simulink library "LumArduinoMAX31856"  (R2024a)
settings: Solver=VariableStepAuto  StartTime=0.0  StopTime=10.0  RelTol=1e-3
undefined symbols (not defined in the file or in its folder): deltaT_s, MAX31856_CJTH_REG_READ, MAX31856_CJTL_REG_READ, MAX31856_CJTO_REG_READ, MAX31856_CJTO_REG_WRITE, MAX31856_CR0_REG_READ, MAX31856_CR0_REG_WRITE, MAX31856_CR1_REG_READ, MAX31856_CR1_REG_WRITE, MAX31856_LTCBH_REG_READ, MAX31856_LTCBL_REG_READ, MAX31856_LTCBM_REG_READ, MAX31856_MASK_REG_WRITE, pin_CS
libraries: arduinolib x12, LumArduino x8
settings Model: Creator=chris  LastModifiedBy=chris

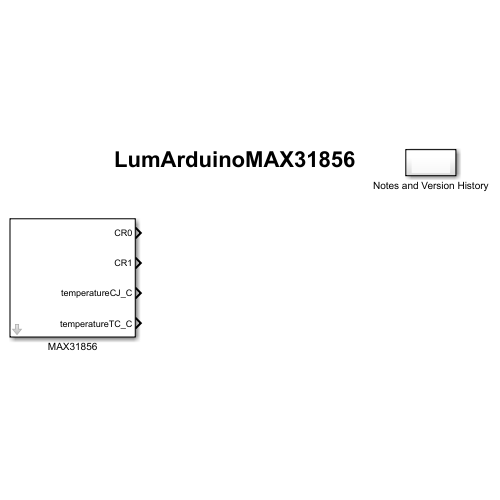
[thumbnail: Simulink's stored preview of the top-level diagram]
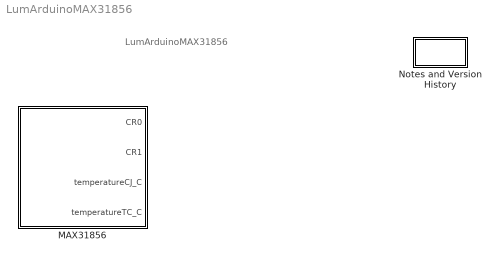
== system LumArduinoMAX31856 ==
  note: LumArduinoMAX31856
  MAX31856 : Subsystem  mask{MAX31856_CR0_REG_READ=MAX31856_CR0_REG_READ, MAX31856_CR0_REG_WRITE=MAX31856_CR0_REG_WRITE, MAX31856_CR1_REG_READ=MAX31856_CR1_REG_READ, MAX31856_CR1_REG_WRITE=MAX31856_CR1_REG_WRITE, MAX31856_MASK_REG_WRITE=MAX31856_MASK_REG_WRITE, MAX31856_CJTO_REG_READ=MAX31856_CJTO_REG_READ, MAX31856_CJTO_REG_WRITE=MAX31856_CJTO_REG_WRITE, MAX31856_CJTH_REG_READ=MAX31856_CJTH_REG_READ, MAX31856_CJTL_REG_READ=MAX31856_CJTL_REG_READ, MAX31856_LTCBH_REG_READ=MAX31856_LTCBH_REG_READ, MAX31856_LTCBM_REG_READ=MAX31856_LTCBM_REG_READ, MAX31856_LTCBL_REG_READ=MAX31856_LTCBL_REG_READ, deltaT_s=deltaT_s, pin_CS=pin_CS}
      mask prompts: MAX31856_CR0_REG_READ "CR0 Read Register Address"; MAX31856_CR0_REG_WRITE "CR0 Write Register Address"; MAX31856_CR1_REG_READ "CR1 Read Register Address"; MAX31856_CR1_REG_WRITE "CR1 Write Register Address"; MAX31856_MASK_REG_WRITE "MASK Write Register Address"; MAX31856_CJTO_REG_READ "CJTO Read Register Address"; MAX31856_CJTO_REG_WRITE "CJTO Write Register Address"; MAX31856_CJTH_REG_READ "CJTH Read Register Address"; MAX31856_CJTL_REG_READ "CJTL Read Register Address"; MAX31856_LTCBH_REG_READ "LTCBH Read Register Address"; MAX31856_LTCBM_REG_READ "LTCBM Read Register Address"; MAX31856_LTCBL_REG_READ "LTCBL Read Register Address"; deltaT_s "Sample Time (sec)"; pin_CS "Chip Select Pin"
      mask help:
      | Interface with a MAX31856 breakout board.
      |
      | Currently this only supports K-type thermocouples.
      |
      | Christopher Lum
      | lum@uw.edu
      mask DialogControl ParameterGroupVar Prompt: CR0
      mask DialogControl Container3 Prompt: CR1
      mask DialogControl Container5 Prompt: MASK
      mask DialogControl Container4 Prompt: CJTO
      mask DialogControl Container6 Prompt: CJTL/CJTH
      mask DialogControl Container7 Prompt: LTCBH/LTCBM/LTCBL
      mask DialogControl Container8 Prompt: Misc.
  Notes and Version History : Subsystem

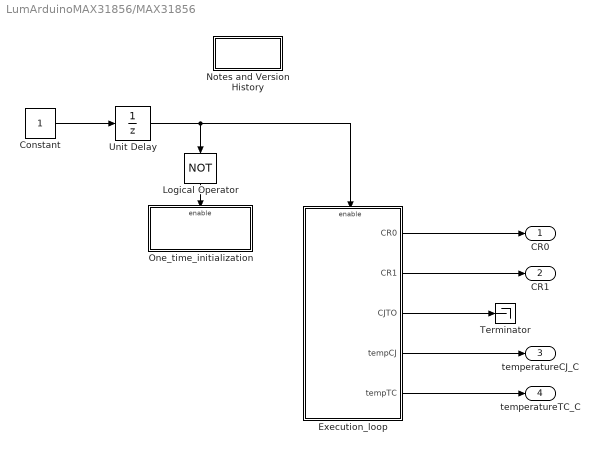
== system LumArduinoMAX31856/MAX31856 ==
  Constant : Constant  OutDataTypeStr=boolean  SampleTime=deltaT_s
  Execution_loop : Subsystem  TreatAsAtomicUnit=on
  Logical Operator : Logic  Operator=NOT  AllPortsSameDT=off  OutDataTypeStr=boolean
  Notes and Version History : Subsystem
  One_time_initialization : Subsystem  TreatAsAtomicUnit=on
  Terminator : Terminator
  Unit Delay : UnitDelay  SampleTime=-1  HasFrameUpgradeWarning=on
  CR0 : Outport
  CR1 : Outport  Port=2
  temperatureCJ_C : Outport  Port=3
  temperatureTC_C : Outport  Port=4
  wires:
  Execution_loop/4(tempCJ) -> temperatureCJ_C/1
  Execution_loop/5(tempTC) -> temperatureTC_C/1
  Execution_loop/3(CJTO) -> Terminator/1
  Execution_loop/2(CR1) -> CR1/1
  Logical Operator/1 -> One_time_initialization/Enable
  Execution_loop/1(CR0) -> CR0/1
  Unit Delay/1 -> Logical Operator/1, Execution_loop/Enable
  Constant/1 -> Unit Delay/1

== system LumArduinoMAX31856/Notes and Version History ==
  note: Interfacing with the MAX31856 sensor
      |
      | Christopher Lum
      | lum@uw.edu
      |
      | Version History
      | 01/04/25: Created

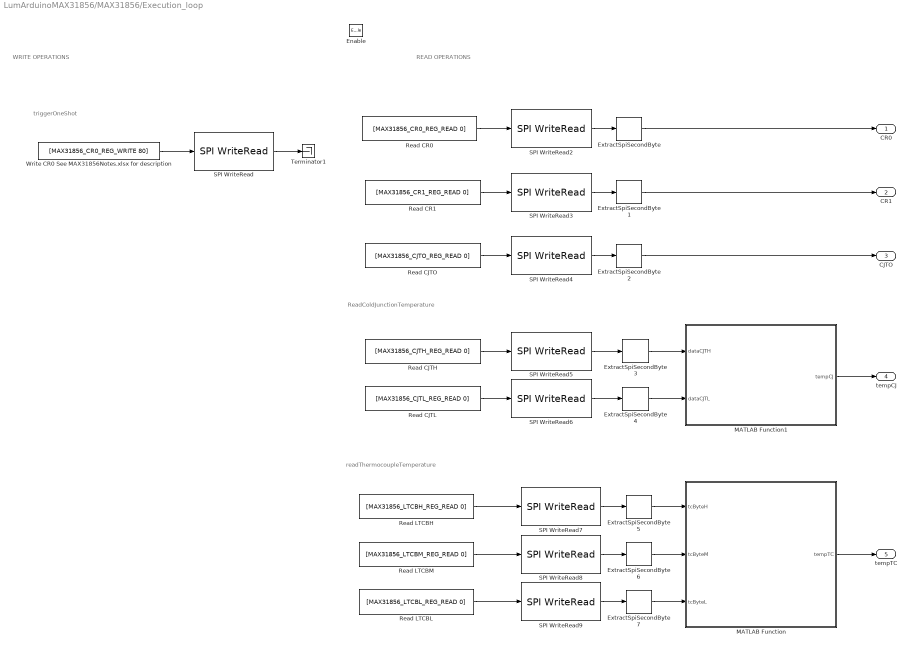
== system LumArduinoMAX31856/MAX31856/Execution_loop ==
  note: triggerOneShot
  note: readThermocoupleTemperature
  note: ReadColdJunctionTemperature
  note: WRITE OPERATIONS
  note: READ OPERATIONS
  Enable : EnablePort  StatesWhenEnabling=reset
  ExtractSpiSecondByte{,1..7} (8 alike) : LumArduino/ExtractSpiSecondByte
  MATLAB Function : MATLAB Function  TreatAsAtomicUnit=on
  MATLAB Function1 : MATLAB Function  TreatAsAtomicUnit=on
  Read CJTH : Constant  Value=[MAX31856_CJTH_REG_READ 0]  OutDataTypeStr=uint8  SampleTime=deltaT_s
  Read CJTL : Constant  Value=[MAX31856_CJTL_REG_READ 0]  OutDataTypeStr=uint8  SampleTime=deltaT_s
  Read CJTO : Constant  Value=[MAX31856_CJTO_REG_READ 0]  OutDataTypeStr=uint8  SampleTime=deltaT_s
  Read CR0 : Constant  Value=[MAX31856_CR0_REG_READ 0]  OutDataTypeStr=uint8  SampleTime=deltaT_s
  Read CR1 : Constant  Value=[MAX31856_CR1_REG_READ 0]  OutDataTypeStr=uint8  SampleTime=deltaT_s
  Read LTCBH : Constant  Value=[MAX31856_LTCBH_REG_READ 0]  OutDataTypeStr=uint8  SampleTime=deltaT_s
  Read LTCBL : Constant  Value=[MAX31856_LTCBL_REG_READ 0]  OutDataTypeStr=uint8  SampleTime=deltaT_s
  Read LTCBM : Constant  Value=[MAX31856_LTCBM_REG_READ 0]  OutDataTypeStr=uint8  SampleTime=deltaT_s
  SPI WriteRead{,2..9} (9 alike) : arduinolib/SPI WriteRead  SPIModule=0  slaveSelectPin_=pin_CS  blockPlatform=arduino
  Terminator1 : Terminator
  Write CR0 See MAX31856Notes.xlsx for description : Constant  Value=[MAX31856_CR0_REG_WRITE 80]  OutDataTypeStr=uint8  SampleTime=deltaT_s
  CR0 : Outport  InitialOutput=0
  CR1 : Outport  Port=2  InitialOutput=0
  CJTO : Outport  Port=3  InitialOutput=0
  tempCJ : Outport  Port=4  InitialOutput=0
  tempTC : Outport  Port=5  InitialOutput=0
  wires:
  Read CR0/1 -> SPI WriteRead2/1
  Read CR1/1 -> SPI WriteRead3/1
  Read CJTO/1 -> SPI WriteRead4/1
  Read CJTH/1 -> SPI WriteRead5/1
  Read CJTL/1 -> SPI WriteRead6/1
  Write CR0 See MAX31856Notes.xlsx for description/1 -> SPI WriteRead/1
  SPI WriteRead/1 -> Terminator1/1
  Read LTCBH/1 -> SPI WriteRead7/1
  Read LTCBM/1 -> SPI WriteRead8/1
  Read LTCBL/1 -> SPI WriteRead9/1
  MATLAB Function1/1(tempCJ) -> tempCJ/1
  MATLAB Function/1(tempTC) -> tempTC/1
  SPI WriteRead2/1 -> ExtractSpiSecondByte/1
  SPI WriteRead3/1 -> ExtractSpiSecondByte1/1
  SPI WriteRead4/1 -> ExtractSpiSecondByte2/1
  ExtractSpiSecondByte/1 -> CR0/1
  ExtractSpiSecondByte1/1 -> CR1/1
  ExtractSpiSecondByte2/1 -> CJTO/1
  SPI WriteRead5/1 -> ExtractSpiSecondByte3/1
  SPI WriteRead6/1 -> ExtractSpiSecondByte4/1
  ExtractSpiSecondByte3/1 -> MATLAB Function1/1(dataCJTH)
  ExtractSpiSecondByte4/1 -> MATLAB Function1/2(dataCJTL)
  SPI WriteRead7/1 -> ExtractSpiSecondByte5/1
  SPI WriteRead8/1 -> ExtractSpiSecondByte6/1
  SPI WriteRead9/1 -> ExtractSpiSecondByte7/1
  ExtractSpiSecondByte5/1 -> MATLAB Function/1(tcByteH)
  ExtractSpiSecondByte6/1 -> MATLAB Function/2(tcByteM)
  ExtractSpiSecondByte7/1 -> MATLAB Function/3(tcByteL)

== system LumArduinoMAX31856/MAX31856/Notes and Version History ==
  note: Interface with a MAX31856 via SPI. This is similar to the functionality outlined in \LumArduinoSDK\Examples\MAX31856\SPI_OneShot\SPI_OneShot.ino except this uses the Simulink Support Package for Arduino Hardware to achieve this functionality.
      |
      | Christopher Lum
      | lum@uw.edu
      |
      | Version History
      | 12/14/24: Created
      | 12/19/24: Continued working
      | 12/20/24: Changed SPI properties via Configuration Parameters > Hardware Implementation > SPI properties
      | 01/04/25: Fixing documentation. Adding support for negative temperatures. Moved to LumArduinoMAX31856.slx library.
      | 01/05/25: Masking block.

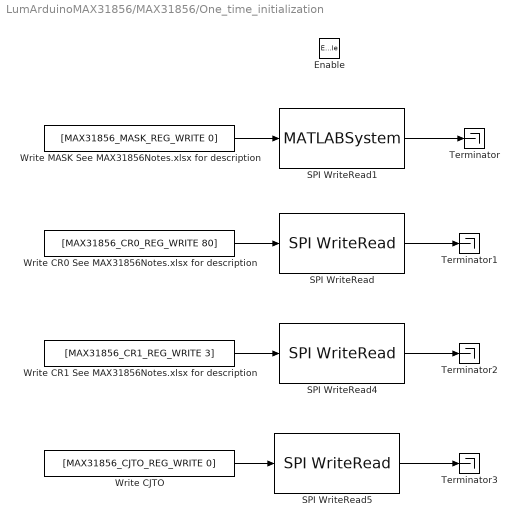
== system LumArduinoMAX31856/MAX31856/One_time_initialization ==
  Enable : EnablePort  StatesWhenEnabling=reset
  SPI WriteRead : arduinolib/SPI WriteRead  SPIModule=0  slaveSelectPin_=pin_CS  blockPlatform=arduino
  SPI WriteRead1 : MATLABSystem  InitFcn=|  System=codertarget.arduinobase.internal.arduinoSPIWriteRead  SPIModule=SPIModule  slaveSelectPin_=slaveSelectPin_  mask(SPI WriteRead){SPIModule=0, slaveSelectPin_=pin_CS, blockPlatform=arduino}
      | codertarget.arduinobase.conflictcheck.validateandregisterBlocks(gcbh);
      | codertarget.arduinobase.blocks.registerSPIBlock(gcbh);
      mask prompts: SPIModule "arduino:blockmask:SPIModuleProp"; slaveSelectPin_ "Chip select (CS) pin"; blockPlatform "Block platform"
      mask help:
      | Write data to and then read data from an SPI device.
      |
      | The block accepts 1-D array of type uint8, uint16, or uint32. The block outputs an array of the same size and data type as the input values.
      mask init:
      | codertarget.arduinobase.blocks.arduinoSPIwriteRead_callback('MaskInitialization');
      settings: LibrarySourceBlock=arduinolib/SPI WriteRead
      mask Help: eval('codertarget.internal.helpView(''arduinoert'', ''arduinolibarduinospiwriteread'')')
      mask TypeOptions SPIModule: SPIModule
      mask TypeOptions slaveSelectPin_: slaveSelectPin_
      mask DialogControl Control2 Prompt: View pin map
      mask DialogControl Control2 Callback:
      | file = [codertarget.arduinobase.internal.getBaseSpPkgRootDir filesep 'blocks' filesep 'mex' filesep 'arduinoPinMapping.html'];
      | web(file)
      mask DialogControl SPIModule Prompt: SPI module
      mask Display:
      | pic=imread('SPIlogo.png');image(pic,[0.32 0.25 0.35 0.55]);text(0.5, 0.15, 'CS pin pin_CS', 'horizontalAlignment', 'center');
      | color('blue');
      | text(0.55, 0.87, 'ARDUINO', 'horizontalAlignment', 'left');
      | color('black');
  SPI WriteRead4 : arduinolib/SPI WriteRead  SPIModule=0  slaveSelectPin_=pin_CS  blockPlatform=arduino
  SPI WriteRead5 : arduinolib/SPI WriteRead  SPIModule=0  slaveSelectPin_=pin_CS  blockPlatform=arduino
  Terminator{,1..3} (4 alike) : Terminator
  Write CJTO : Constant  Value=[MAX31856_CJTO_REG_WRITE 0]  OutDataTypeStr=uint8  SampleTime=deltaT_s
  Write CR0 See MAX31856Notes.xlsx for description : Constant  Value=[MAX31856_CR0_REG_WRITE 80]  OutDataTypeStr=uint8  SampleTime=deltaT_s
  Write CR1 See MAX31856Notes.xlsx for description : Constant  Value=[MAX31856_CR1_REG_WRITE 3]  OutDataTypeStr=uint8  SampleTime=deltaT_s
  Write MASK See MAX31856Notes.xlsx for description : Constant  Value=[MAX31856_MASK_REG_WRITE 0]  OutDataTypeStr=uint8  SampleTime=deltaT_s
  wires:
  SPI WriteRead/1 -> Terminator1/1
  Write CR0 See MAX31856Notes.xlsx for description/1 -> SPI WriteRead/1
  Write CR1 See MAX31856Notes.xlsx for description/1 -> SPI WriteRead4/1
  SPI WriteRead4/1 -> Terminator2/1
  SPI WriteRead5/1 -> Terminator3/1
  Write CJTO/1 -> SPI WriteRead5/1
  Write MASK See MAX31856Notes.xlsx for description/1 -> SPI WriteRead1/1
  SPI WriteRead1/1 -> Terminator/1

== matlab function LumArduinoMAX31856/MAX31856/Execution_loop/MATLAB Function ==
  data: tcByteH input; tempTC output; tcByteM input; tcByteL input
function tempTC = readThermocoupleTemperature(tcByteH,tcByteM,tcByteL)

ret = int32(tcByteH);

ret = bitshift(ret,8);
ret = bitor(ret,int32(tcByteM));
ret = bitshift(ret,8);
ret = bitor(ret,int32(tcByteL));

temp24 = ret;

%check if value is negative or not
if(BitIs1(tcByteH,7))
    %pad the left 8 bits with 1s
    B_int32 = int32(-16777216);
    
    %-16777216 as an int32 has the bit pattern of 0xFF000000
    temp24 = bitor(temp24,B_int32);
end

%perform conversion (bottom 5 bits are unused)
temp24 = bitshift(temp24,-5);

tempTC = double(temp24)*0.0078125;

== matlab function LumArduinoMAX31856/MAX31856/Execution_loop/MATLAB Function1 ==
  data: dataCJTH input; tempCJ output; dataCJTL input
function tempCJ = readColdJunctionTemperature(dataCJTH,dataCJTL)

ret = int16(dataCJTH);

ret = bitshift(ret,8);
ret = bitor(ret,int16(dataCJTL));

tempCJ = double(ret)/256;
